simulink model "x1_2"  (R2025b)
settings: Solver=ode4  StartTime=0.0  StopTime=T_SIMULATION  FixedStep=0.001  RelTol=1e-3
values from neighbouring files (symbols this model uses):
  d = 0.165    [live_script.m]    (also in script_1_1.m; script_1_simulation.m; script_2_motion_planning.m)
  Q_INITIAL = [1;1;0]    [live_script.m]    (also in script_1_1.m = [0;0;0]; script_1_simulation.m)
  r = 0.03    [live_script.m]    (also in script_1_1.m; script_1_simulation.m; script_2_motion_planning.m)
  v = 0    [live_script.m]    (also in script_1_1.m = 5; script_1_simulation.m)
  v1_chained = 10    [script_1_1.m]
  v2_chained = 10    [script_1_1.m]
  w = 2.0    (= 2)    [live_script.m]    (also in script_1_1.m = 10; script_1_simulation.m)
  Z_INITIAL = [0;0;0]    [script_1_1.m]
settings Model: Creator=alber  LastModifiedBy=llp

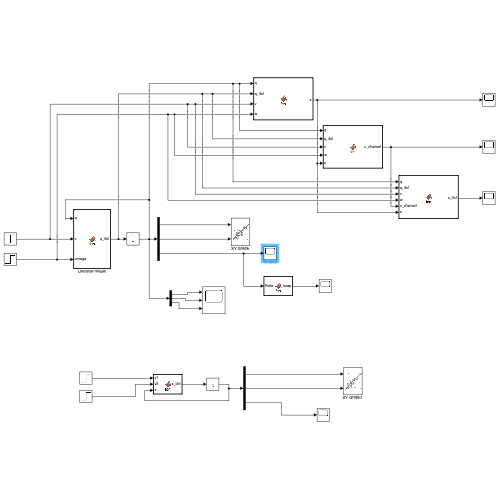
[thumbnail: Simulink's stored preview of the top-level diagram]
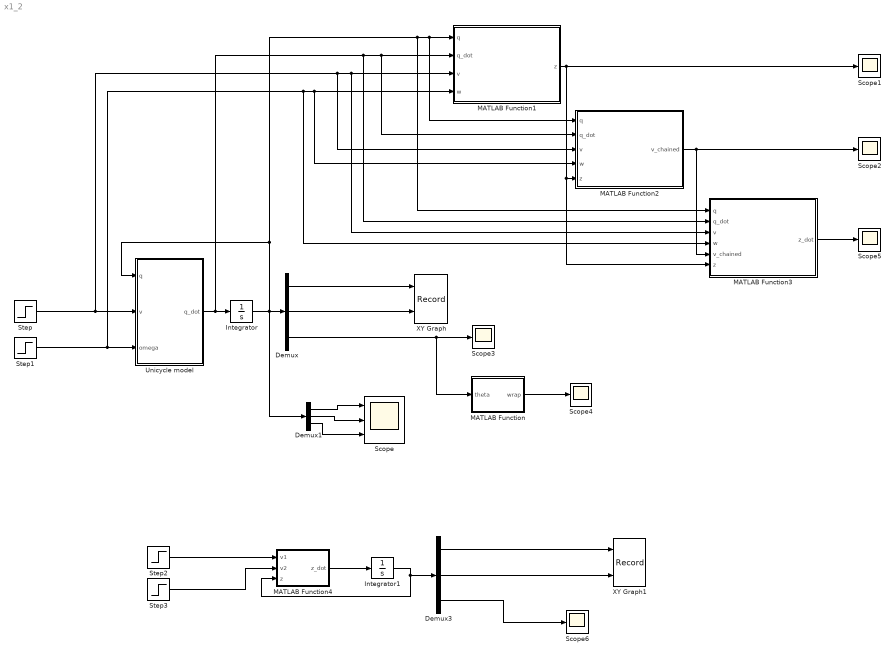
== system x1_2 ==
  Demux : Demux  Outputs=3
  Demux1 : Demux  Outputs=3
  Demux3 : Demux  Outputs=3
  Integrator : Integrator  InitialCondition=Q_INITIAL
  Integrator1 : Integrator  InitialCondition=Z_INITIAL
  MATLAB Function : MATLAB Function  TreatAsAtomicUnit=on
  MATLAB Function1 : MATLAB Function  TreatAsAtomicUnit=on
  MATLAB Function2 : MATLAB Function  TreatAsAtomicUnit=on
  MATLAB Function3 : MATLAB Function  TreatAsAtomicUnit=on
  MATLAB Function4 : MATLAB Function  TreatAsAtomicUnit=on
  Scope : Scope  NumInputPorts=3
      settings: ActiveDisplayYMinimum=-18.558005528495297  ActiveDisplayYMaximum=3.3856861200938342
  Scope{1..6} (6 alike) : Scope
      Scope1 settings: ActiveDisplayYMinimum=-11.812707544351312  ActiveDisplayYMaximum=101.31437491234547
      Scope2 settings: ActiveDisplayYMinimum=-1  ActiveDisplayYMaximum=1  DataLoggingVariableName=ScopeData2
      Scope3 settings: ActiveDisplayYMinimum=-11.250208333334474  ActiveDisplayYMaximum=101.25187500001027  DataLoggingVariableName=ScopeData3
      Scope4 settings: DataLoggingVariableName=ScopeData4
      Scope5 settings: ActiveDisplayYMinimum=-6.8749921721339424  ActiveDisplayYMaximum=11.874999130237105  DataLoggingVariableName=ScopeData5
      Scope6 settings: ActiveDisplayYMinimum=-1  ActiveDisplayYMaximum=1  DataLoggingVariableName=ScopeData6
  Step : Step  After=v  SampleTime=0
  Step1 : Step  After=w  SampleTime=0
  Step2 : Step  After=v1_chained  SampleTime=0
  Step3 : Step  After=v2_chained  SampleTime=0
  Unicycle model : MATLAB Function  TreatAsAtomicUnit=on
  XY Graph : Record  NumPorts=2.0  FileSettingsInternal="{\"entries\":[{\"content\":{\"excelSettings\":{\"content\":{},\"type\":\"Streamout.ExcelSettings\"},\"parquetSettings\":{\"content\":{},\"type\":\"Streamout.ParquetSettings\"}},\"type\":\"Streamout.FileSettingStorage\",\"uuid\":\"\"}],\"packageUris\":[\"http:\\/\\/schema.mathworks.com\\/mf0\\/streamout_blocks\\/R2020a\"],\"version\":\"1.0\"}"  FrameSettings=[0, 0]  Layout=[1 1]  SignalsInternal="{\"entries\":[{\"content\":{\"signals\":[{\"content\":{\"blockPath\":[],\"dimensions\":[1,1],\"domain\":\"\",\"lineColor\":\"#a2142f\",\"plots\":[ 1 ],\"port\":1,\"sid\":[\"\"],\"signalID\":1,\"signalName\":\"Demux:1\"},\"type\":\"RecordBlkView.Signal\",\"uuid\":\"\"},{\"content\":{\"blockPath\":[],\"dimensions\":[1,1],\"domain\":\"\",\"lineColor\":\"#139fff\",\"plots\":[ 1 ],\"port\":2,\"sid\":[\"\"],\"signalID\":2,\"signalName\":\"Demux:2\"},\"type\":\"RecordBlkView.Signal\",\"uuid\":\"\"}]},\"type\":\"RecordBlkView.InputSignals\",\"uuid\":\"\"}],\"packageUris\":[\"http:\\/\\/schema.mathworks.com\\/mf0\\/streamout_blocks\\/R2020a\"],\"version\":\"1.0\"}"  VisualizationBindings="{\"xyplotplugin\":{\"info\":[{\"series\":[{\"bindingParametersList\":[{\"parameter\":\"X-Axis\",\"signalID\":1,\"signalName\":\"Demux:1\"},{\"parameter\":\"Y-Axis\",\"signalID\":2,\"signalName\":\"Demux:2\"}],\"seriesID\":0}],\"subplotID\":1}]}}"  CompatibilityTag=XY
  XY Graph1 : Record  NumPorts=2.0  FileSettingsInternal="{\"entries\":[{\"content\":{\"excelSettings\":{\"content\":{},\"type\":\"Streamout.ExcelSettings\"},\"parquetSettings\":{\"content\":{},\"type\":\"Streamout.ParquetSettings\"}},\"type\":\"Streamout.FileSettingStorage\",\"uuid\":\"\"}],\"packageUris\":[\"http:\\/\\/schema.mathworks.com\\/mf0\\/streamout_blocks\\/R2020a\"],\"version\":\"1.0\"}"  FrameSettings=[0, 0]  Layout=[1 1]  SignalsInternal="{\"entries\":[{\"content\":{\"signals\":[{\"content\":{\"blockPath\":[],\"dimensions\":[1,1],\"domain\":\"\",\"lineColor\":\"#a2142f\",\"plots\":[ 1 ],\"port\":1,\"sid\":[\"\"],\"signalID\":1,\"signalName\":\"Demux3:1\"},\"type\":\"RecordBlkView.Signal\",\"uuid\":\"\"},{\"content\":{\"blockPath\":[],\"dimensions\":[1,1],\"domain\":\"\",\"lineColor\":\"#139fff\",\"plots\":[ 1 ],\"port\":2,\"sid\":[\"\"],\"signalID\":2,\"signalName\":\"Demux3:2\"},\"type\":\"RecordBlkView.Signal\",\"uuid\":\"\"}]},\"type\":\"RecordBlkView.InputSignals\",\"uuid\":\"\"}],\"packageUris\":[\"http:\\/\\/schema.mathworks.com\\/mf0\\/streamout_blocks\\/R2020a\"],\"version\":\"1.0\"}"  VisualizationBindings="{\"xyplotplugin\":{\"info\":[{\"series\":[{\"bindingParametersList\":[{\"parameter\":\"X-Axis\",\"signalID\":1,\"signalName\":\"Demux3:1\"},{\"parameter\":\"Y-Axis\",\"signalID\":2,\"signalName\":\"Demux3:2\"}],\"seriesID\":0}],\"subplotID\":1}]}}"  CompatibilityTag=XY
  wires:
  Unicycle model/1(q_dot) -> MATLAB Function3/2(q_dot), MATLAB Function2/2(q_dot), MATLAB Function1/2(q_dot), Integrator/1
  Integrator/1 -> Demux1/1, Demux/1, MATLAB Function3/1(q), MATLAB Function2/1(q), MATLAB Function1/1(q), Unicycle model/1(q)
  Demux/2 -> XY Graph/2
  Demux/1 -> XY Graph/1
  Demux1/1 -> Scope/1
  Demux1/2 -> Scope/2
  Demux1/3 -> Scope/3
  Demux/3 -> MATLAB Function/1(theta), Scope3/1
  MATLAB Function/1(wrap) -> Scope4/1
  Step/1 -> MATLAB Function2/3(v), MATLAB Function3/3(v), MATLAB Function1/3(v), Unicycle model/2(v)
  Step1/1 -> MATLAB Function3/4(w), MATLAB Function2/4(w), MATLAB Function1/4(w), Unicycle model/3(omega)
  MATLAB Function1/1(z) -> Scope1/1, MATLAB Function3/6(z), MATLAB Function2/5(z)
  MATLAB Function2/1(v_chained) -> Scope2/1, MATLAB Function3/5(v_chained)
  MATLAB Function3/1(z_dot) -> Scope5/1
  Step2/1 -> MATLAB Function4/1(v1)
  Step3/1 -> MATLAB Function4/2(v2)
  MATLAB Function4/1(z_dot) -> Integrator1/1
  Integrator1/1 -> Demux3/1, MATLAB Function4/3(z)
  Demux3/1 -> XY Graph1/1
  Demux3/2 -> XY Graph1/2
  Demux3/3 -> Scope6/1

== matlab function x1_2/Unicycle model ==
  data: q input; v input; q_dot output; omega input; r parameter; d parameter
function q_dot = fcn(q, v, omega, r, d)
%write the unicycle model
q_dot= zeros(3,1);

q_dot(1) = v*cos(q(3));
q_dot(2) = v*sin(q(3));
q_dot(3) = omega;

== matlab function x1_2/MATLAB Function1 ==
  data: q input; z output; q_dot input; v input; w input
function z = fcn(q,q_dot,v,w)

z = zeros(3,1);
z(1)= q(3);
z(2)= q(1)*cos(q(3))+q(2)*sin(q(3));
z(3) = q(1)*sin(q(3))-q(2)*cos(q(3));

== matlab function x1_2/MATLAB Function ==
  data: theta input; wrap output
function wrap = fcn(theta)

wrap = mod(theta+pi,2*pi)-pi ;

== matlab function x1_2/MATLAB Function2 ==
  data: q input; v_chained output; q_dot input; v input; w input; z input
function v_chained = fcn(q,q_dot,v,w,z)


v_chained = zeros(2,1);
v_chained(1) = w;
v_chained(2) = v-z(3)*w;

== matlab function x1_2/MATLAB Function3 ==
  data: q input; z_dot output; q_dot input; v input; w input; v_chained input; z input
function z_dot = fcn(q,q_dot,v,w,v_chained,z)


z_dot = zeros(3,1);
z_dot(1) = v_chained(1);
z_dot(2) = v_chained(2);
z_dot(3) = z(2)*v_chained(1);

== matlab function x1_2/MATLAB Function4 ==
  data: v1 input; z_dot output; v2 input; z input
function z_dot = fcn(v1,v2,z)

z_dot = zeros(3,1);
z_dot(1)= v1;
z_dot(2)= v2;
z_dot(3) = z(2)*v1;
